simulink model "USV"  (R2022a)
settings: Solver=ode4  StartTime=0.0  StopTime=inf  FixedStep=0.001  RelTol=1e-3
PreLoadFcn:
  | [filepath,name,ext]  = fileparts(get_param(bdroot, 'FileName'));
  | InitFileName=[name,'_init.m'];
  | cd(filepath);
InitFcn:
  | [filepath,name,ext]  = fileparts(get_param(bdroot, 'FileName'));
  | InitFileName=[name,'_init.m'];
  | cd(filepath);
  | try
  | run(InitFileName);
  | end
values from neighbouring files (symbols this model uses):
  BoatParam_cf = 0.1    [USV_init.m]
  BoatParam_cg = 0.1    [USV_init.m]
  BoatParam_len = 1.5    [USV_init.m]
  BoatParam_lenSlope = pi/6    (= 0.523598775598)    [USV_init.m]
  BoatParam_waterDensity = 1000    [USV_init.m]
  BoatParam_widSlope = pi/4    (= 0.785398163397)    [USV_init.m]
  BoatParam_width = 0.8    [USV_init.m]
  ModelPara_coborigin = [0;0;0]    [USV_init.m]
  ModelParam_envAltitude = -600    [USV_init.m]
  ModelParam_GPSEphFinal = 0.3    [USV_init.m]
  ModelParam_GPSEpvFinal = 0.4    [USV_init.m]
  ModelParam_noiseGPSSampTime = 0.2    [USV_init.m]
  ModelParam_noisePowerOffGainAccel = 0.04    [USV_init.m]
  ModelParam_noisePowerOffGainAccelZ = 0.03    [USV_init.m]
  ModelParam_noisePowerOffGainGyro = 0.02    [USV_init.m]
  ModelParam_noisePowerOffGainGyroZ = 0.025    [USV_init.m]
  ModelParam_noisePowerOffGainMag = 0.02    [USV_init.m]
  ModelParam_noisePowerOffGainMagZ = 0.035    [USV_init.m]
  ModelParam_noisePowerOnGainAccel = 0.8    [USV_init.m]
  ModelParam_noisePowerOnGainAccelZ = 4.5    [USV_init.m]
  ModelParam_noisePowerOnGainGyro = 2    [USV_init.m]
  ModelParam_noisePowerOnGainGyroZ = 1    [USV_init.m]
  ModelParam_noisePowerOnGainMag = 0.025    [USV_init.m]
  ModelParam_noisePowerOnGainMagZ = 0.05    [USV_init.m]
  ModelParam_noiseUpperGPS = 0.5    [USV_init.m]
  ModelParam_uavCCm = [1 1 1]*200    [USV_init.m]
  ModelParam_uavCd = [2 200 200]    [USV_init.m]
  ModelParam_uavDearo = -0    (= 0)    [USV_init.m]
  ModelParam_uavMass = 227    [USV_init.m]
  ModelParam_uavType = int16(608)    [USV_init.m]
  motor = [motor,motorTmp]    [USV_init.m]
undefined symbols (not defined in the file or in its folder): Earth, ModelParam_GPSEpvInitial, ModelParam_GPSEpvTimeConstant, ModelParam_timeSamp, Newton, Raphson, USVPara, WGS84
libraries: RflySimModelLab x8, FaultUSVModelLib x4, aerolibtransform2 x4, vrlib x4, sharedutil x3, aerolibasang x3, sharedtransform x2, shared6dof x1, aerolibatmos2 x1, aerolibconvert2 x1, aerolibobsolete x1, simulink x1
(part 1 of 2)
settings Model: SimulationMode=accelerator  Creator=Jinrui  LastModifiedBy=dream
settings SolverCC: AlgebraicLoopSolver=TrustRegion
settings DataIOCC: ReturnWorkspaceOutputs=off
settings OptimizationCC: ZeroExternalMemoryAtStartup=off  ZeroInternalMemoryAtStartup=off  EfficientTunableParamExpr=on
settings DebuggingCC: ParameterTunabilityLossMsg=error  UnconnectedInputMsg=warning  UnconnectedOutputMsg=warning  UnconnectedLineMsg=warning  SFMachineParentedDataDiag=warning  ArithmeticOperatorsInVariantConditions=warning
settings SFSimCC: SimUseLocalCustomCode=off  MATLABDynamicMemAlloc=off  CustomCodeUndefinedFunction=UseInterfaceOnly  SimTargetLang=C++
settings RTWCC: SystemTargetFile=ert.tlc  GenCodeOnly=on  GenerateMakefile=off  PackageGeneratedCodeAndArtifacts=on  PackageName=MulticopterModel  TemplateMakefile=ert_default_tmf  RTWUseLocalCustomCode=off  TargetLang=C++  RTWCompilerOptimization=on
settings CodeAppCC: ForceParamTrailComments=on  OperatorAnnotations=on  SimulinkDataObjDesc=on  SFDataObjDesc=on  MATLABFcnDesc=on  InsertBlockDesc=on  StateflowObjectComments=on  MATLABSourceComments=on
settings ERTTargetCC: TargetLangStandard=C++03 (ISO)  MultiwordLength=2048  GenerateSampleERTMain=on  CodeInterfacePackaging=C++ class  SupportContinuousTime=on  MultiInstanceErrorCode=None  RootIOFormat=Structure reference  ERTCustomFileTemplate=example_file_process.tlc  ERTFilePackagingFormat=Compact
settings SimscapeCC: SimscapeNormalizeSystem=off

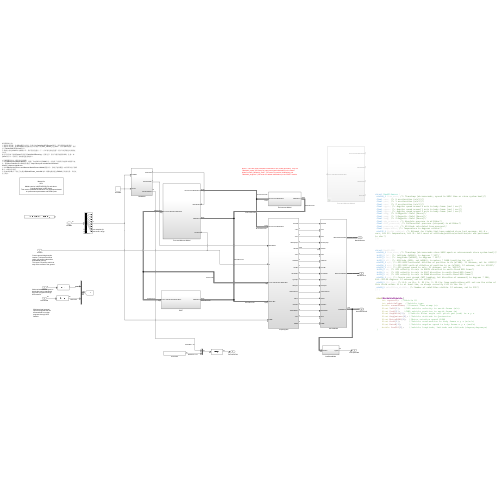
[thumbnail: Simulink's stored preview of the top-level diagram]
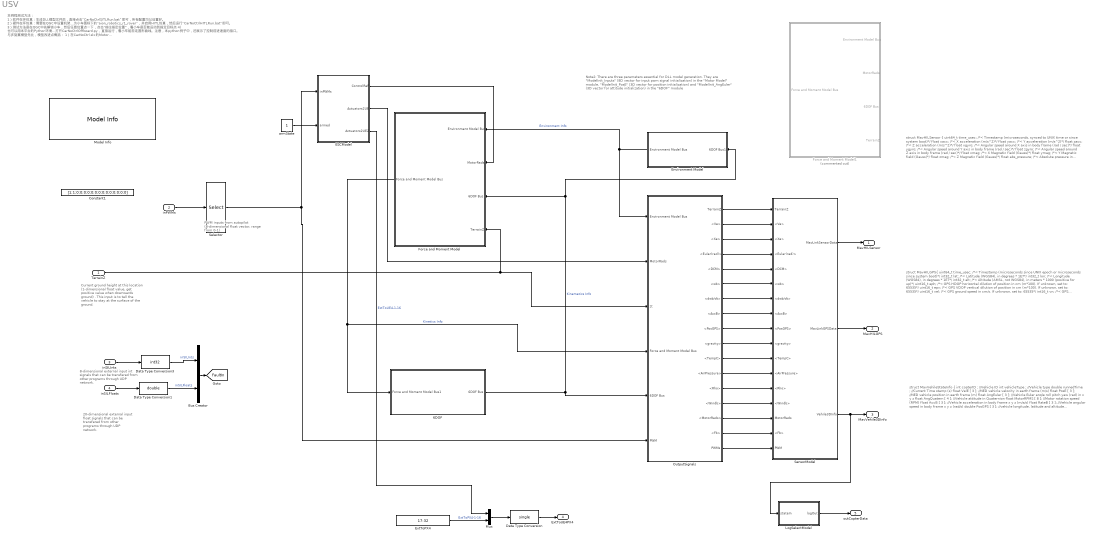
== system USV ==
  note: PWM inputs from autopilot (8-dimensional float vector, range from 0-1)
  note: Note2: There are three parameters essential for DLL model generation. They are "ModelInit_Inputs" (8D vector for input pwm signal initialization) in the "Motor Model" module, "ModelInit_PosE" (3D vector for position initialization) and "ModelInit_AngEuler" (3D vector for attitude initialization) in the "6DOF" module
  note: Current ground height at this location (1-dimensional float value, get positive value when downwards ground) .
      | This input is to tell the vehicle to stay at the surface of the ground.
  note: 本例程测试方法：
      | 1）软件在环仿真：生成DLL模型文件后，直接点击“CarNoCtrlSITLRun.bat”即可，所有配置均以设置好。
      | 2）硬件在环仿真：需要在QGC中设置机架为小车图标下的“aion_robotics_r1_rover”，并启用HITL仿真，然后运行“CarNoCtrlHITLRun.bat”即可。
      | 3）测试方法是在QGC中先解锁小车，然后任意位置点一下，点击"前往指定位置"，看小车是否能运动到指定目标点
      | 4) 也可以用本平台的Python环境打开CarNoCtrlOffboard.py，直接运行，看小车能否走圆形曲线。注意，本python例子中，还展示了控制前进速度的接口。
      |
      | 与多旋翼模型先比，模型改进点概括：
      | 1）在CarNoCtrl.slx的Motor Model中，设置了只响应0和1号PWM信号，分别给了左侧两个电机和右侧两个电机，遵循Aion Robotics R1 UGV机架模式。https://docs.px4.io/master/en/airframes/airframe_reference.html#rover
      | 2）在CarNoCtrl.slx的Force and Moment Model/Ground Model模型中个，修改了地面模型，响应四个轮子的摩擦力，来驱动车前进。
      | 3）在init.m参数中，设定了电机参数ModelParam_motorWb为0，确保电机转速与PWM成正比例关系，从而支持正反转。
  note: struct MavHILGPS{
      | uint64_t time_usec; /*< Timestamp (microseconds since UNIX epoch or microseconds since system boot)*/
      | int32_t lat; /*< Latitude (WGS84), in degrees * 1E7*/
      | int32_t lon; /*< Longitude (WGS84), in degrees * 1E7*/
      | int32_t alt; /*< Altitude (AMSL, not WGS84), in meters * 1000 (positive for up)*/
      | uint16_t eph; /*< GPS HDOP horizontal dilution of position in cm (m*100). If unknown, set to: 65535*/
      | uint16_t epv; /*< GPS VDOP vertical dilution of position in cm (m*100). If unknown, set to: 65535*/
      | uint16_t vel; /*< GPS ground speed in cm/s. If unknown, set to: 65535*/
      | int16_t vn; /*< GPS velocity in cm/s in NORTH direction in earth-fixed NED frame*/
      | int16_t ve; /*< GPS velocity in cm/s in EAST direction in earth-fixed NED frame*/
      | int16_t vd; /*< GPS velocity in cm/s in DOWN direction in earth-fixed NED frame*/
      | uint16_t cog; /*< Course over ground (NOT heading, but direction of movement) in degrees * 100, 0.0..359.99 degrees. If unknown, set to: 65535*/
      | uint8_t fix_type; /*< 0-1: no fix, 2: 2D fix, 3: 3D fix. Some applications will not use the value of this field unless it is at least two, so always correctly fill in the fix.*/
      | uint8_t satellites_visible; /*< Number of satellites visible. If unknown, set to 255*/
      | }) ;
  note: struct MavHILSensor {
      | uint64_t time_usec; /*< Timestamp (microseconds, synced to UNIX time or since system boot)*/
      | float xacc; /*< X acceleration (m/s^2)*/
      | float yacc; /*< Y acceleration (m/s^2)*/
      | float zacc; /*< Z acceleration (m/s^2)*/
      | float xgyro; /*< Angular speed around X axis in body frame (rad / sec)*/
      | float ygyro; /*< Angular speed around Y axis in body frame (rad / sec)*/
      | float zgyro; /*< Angular speed around Z axis in body frame (rad / sec)*/
      | float xmag; /*< X Magnetic field (Gauss)*/
      | float ymag; /*< Y Magnetic field (Gauss)*/
      | float zmag; /*< Z Magnetic field (Gauss)*/
      | float abs_pressure; /*< Absolute pressure in millibar*/
      | float diff_pressure; /*< Differential pressure (airspeed) in millibar*/
      | float pressure_alt; /*< Altitude calculated from pressure*/
      | float temperature; /*< Temperature in degrees celsius*/
      | uint32_t fields_updated; /*< Bitmask for fields that have updated since last message, bit 0 = xacc, bit 12: temperature, bit 31: full reset of attitude/position/velocities/etc was performed in sim.*/
      | });
  note: struct MavVehileStateInfo {
      | int copterID ; //Vehicle ID
      | int vehicleType ; //Vehicle type
      | double runnedTime ; //Current Time stamp (s)
      | float VelE [ 3 ]; //NED vehicle velocity in earth frame (m/s)
      | float PosE [ 3 ]; //NED vehicle position in earth frame (m)
      | float AngEuler [ 3 ]; //Vehicle Euler angle roll pitch yaw (rad) in x y z
      | float AngQuatern [ 4 ]; //Vehicle attitude in Quaternion
      | float MotorRPMS [ 8 ]; //Motor rotation speed (RPM)
      | float AccB [ 3 ]; //Vehicle acceleration in body frame x y z (m/s/s)
      | float RateB [ 3 ]; //Vehicle angular speed in body frame x y z (rad/s)
      | double PosGPS [ 3 ]; //vehicle longitude, latitude and altitude (degree,degree,m)
      | }
  note: 20-dimensional external input float signals that can be transfered from other programs through UDP network.
  note: 8-dimensional external input int signals that can be transfered from other programs through UDP network.
  TerrainZ : Inport
  inPWMs : Inport  Port=2
  inSILInts : Inport  Port=3  OutDataTypeStr=int32  PortDimensions=8
  inSILFloats : Inport  Port=4  OutDataTypeStr=single  PortDimensions=20
  6DOF : Subsystem
  Bus Creator : BusCreator  Inputs=2
  Constant1 : Constant  Value=[1;1;0;0;0;0;0;0;0;0;0;0;0;0;0;0]
  Data Type Conversion : DataTypeConversion  OutDataTypeStr=single  SaturateOnIntegerOverflow=off  RndMeth=Floor
  Data Type Conversion1 : DataTypeConversion  OutDataTypeStr=double  SaturateOnIntegerOverflow=off  RndMeth=Floor
  Data Type Conversion3 : DataTypeConversion  OutDataTypeStr=int32  SaturateOnIntegerOverflow=off  RndMeth=Floor
  ESCModel : Subsystem
  Environment Model : Subsystem
  ExtToPX4 : Constant  Value=17:32
  Force and Moment Model : Subsystem
  Force and Moment Model1 : Subsystem  Commented=on
  LogSelectModel : Subsystem
  Model Info : simulink/Model-Wide Utilities/Model Info  Frame=on  DisplayStringWithTags=|  HorizontalTextAlignment=Center  LeftAlignmentValue=0.5
      | Model Info
      | %<ModelName> 
      | %<Description>   
      | Matlab version is MATLAB R2017b and above. 
      | Coordinate frame is NED frame.
      |  This model  simulates the behavior of a multicopters based 
      | on performance parameters and RPM inputs
  Mux : Mux  Inputs=2
  OutputSignals : Subsystem
  Selector : Selector  InputPortWidth=16  IndexOptions=Index vector (dialog)  Indices=[1:8]  OutputSizes=1
  SensorModel : Subsystem
  armState : Constant
  MavHILSensor : Outport  OutDataTypeStr=Bus: MavLinkSensor  VectorParamsAs1DForOutWhenUnconnected=off
  MavHILGPS : Outport  Port=2  OutDataTypeStr=Bus: MavLinkGPS  VectorParamsAs1DForOutWhenUnconnected=off
  MavVehile3DInfo : Outport  Port=3  OutDataTypeStr=Bus: MavVehileInfo  VectorParamsAs1DForOutWhenUnconnected=off
  ExtToUE4PX4 : Outport  Port=4  OutDataTypeStr=single  PortDimensions=32  VectorParamsAs1DForOutWhenUnconnected=off
  outCopterData : Outport  Port=5  OutDataTypeStr=double  PortDimensions=32  VectorParamsAs1DForOutWhenUnconnected=off
  tag scope: FaultIn=global
  wires:
  OutputSignals/9(<PosGPS>) -> SensorModel/9(<PosGPS>)
  Environment Model/1(Environment Model Bus) -> Force and Moment Model/1(Environment Model Bus), OutputSignals/1(Environment Model Bus)  "Environment Info"
  OutputSignals/3(<Xe>) -> SensorModel/3(<Xe>)
  SensorModel/1(MavLinkSensorData) -> MavHILSensor/1
  OutputSignals/15(<MotorRads>) -> SensorModel/15(MotorRads)
  OutputSignals/12(<AirPressure>) -> SensorModel/12(<AirPressure>)
  Data Type Conversion/1 -> ExtToUE4PX4/1
  Selector/1 -> OutputSignals/6(PWM), ESCModel/1(inPWMs)
  OutputSignals/17(PWMs) -> SensorModel/17(PWM)
  OutputSignals/4(<Eular(rad)>) -> SensorModel/4(<Eular(rad)>)
  OutputSignals/2(<Ve>) -> SensorModel/2(<Ve>)
  OutputSignals/13(<Rho>) -> SensorModel/13(<Rho>)
  OutputSignals/8(<AccB>) -> SensorModel/8(<AccB>)
  SensorModel/3(Vehile3DInfo) -> LogSelectModel/1(stateIn), MavVehile3DInfo/1
  inPWMs/1 -> Selector/1
  SensorModel/2(MavLinkGPSData) -> MavHILGPS/1
  OutputSignals/16(<Fb>) -> SensorModel/16(<Fb>)
  ESCModel/2(Actuators2UE) -> OutputSignals/2(MotorRads)
  OutputSignals/1(TerrainZ) -> SensorModel/1(TerrainZ)
  TerrainZ/1 -> Force and Moment Model/4(TerrainZ), OutputSignals/3(zt)
  OutputSignals/10(<gravity>) -> SensorModel/10(<gravity>)
  OutputSignals/6(<wb>) -> SensorModel/6(<wb>)
  OutputSignals/14(<Windb>) -> SensorModel/14(<Windb>)
  OutputSignals/5(<DCM>) -> SensorModel/5(<DCM>)
  Mux/1 -> Data Type Conversion/1
  ExtToPX4/1 -> Mux/2  "ExtToPX4-1-16"
  ESCModel/1(ControlRef) -> Force and Moment Model/2(MotorRads)
  OutputSignals/11(<TempC>) -> SensorModel/11(<TempC>)
  ESCModel/3(Actuators2UE2) -> Mux/1  "ExtToUE4-1-16"
  6DOF/1(6DOF Bus) -> Environment Model/1(6DOF Bus1), Force and Moment Model/3(6DOF Bus), OutputSignals/5(6DOF Bus)  "Kinematics Info"
  OutputSignals/7(<dwb/dt>) -> SensorModel/7(<dwb/dt>)
  Force and Moment Model/1(Force and Moment Model Bus) -> OutputSignals/4(Force and Moment Model Bus), 6DOF/1(Force and Moment Model Bus1)  "Kinetics Info"
  armState/1 -> ESCModel/2(armed)
  Data Type Conversion1/1 -> Bus Creator/2  "inSILFloats"
  Bus Creator/1 -> [FaultIn]
  Data Type Conversion3/1 -> Bus Creator/1  "inSILInts"
  LogSelectModel/1(logOut) -> outCopterData/1
  inSILInts/1 -> Data Type Conversion3/1
  inSILFloats/1 -> Data Type Conversion1/1

== system USV/6DOF ==
  Force and Moment Model Bus1 : Inport
  Bus Creator : BusCreator  Inputs=8
  Bus Selector2 : BusSelector  OutputSignals=Fb,Mb
  Custom Variable Mass 6DOF (Quaternion) : shared6dof/6DOF (Euler Angles)  units=Metric (MKS)  mtype=Fixed  rep=Quaternion  xme_0=ModelInit_PosE  Vm_0=ModelInit_VelB  eul_0=ModelInit_AngEuler  pm_0=ModelInit_RateB  mass_0=ModelParam_uavMass  mass_e=0.5  mass_f=2.0  inertia=ModelParam_uavJ  inertia_e=eye(3)  inertia_f=2*eye(3)  k_quat=1.0  vre_flag=off  abi_flag=off  aMode=aMode  xme_statename=''  Vm_statename=''  eul_statename=''  quat_statename=''  pm_statename=''  mass_statename=''
      settings: SourceProductBaseCode=AE,PW,DR,MT,VE
  6DOF Bus : Outport  VectorParamsAs1DForOutWhenUnconnected=off
  wires:
  Custom Variable Mass 6DOF (Quaternion)/8 -> Bus Creator/8  "AccB"
  Custom Variable Mass 6DOF (Quaternion)/5 -> Bus Creator/5  "Vb"
  Custom Variable Mass 6DOF (Quaternion)/6 -> Bus Creator/6  "wb"
  Custom Variable Mass 6DOF (Quaternion)/1 -> Bus Creator/1  "Ve"
  Custom Variable Mass 6DOF (Quaternion)/4 -> Bus Creator/4  "DCM"
  Custom Variable Mass 6DOF (Quaternion)/2 -> Bus Creator/2  "Xe"
  Custom Variable Mass 6DOF (Quaternion)/3 -> Bus Creator/3  "Eular(rad)"
  Custom Variable Mass 6DOF (Quaternion)/7 -> Bus Creator/7  "dwb/dt"
  Bus Creator/1 -> 6DOF Bus/1
  Force and Moment Model Bus1/1 -> Bus Selector2/1
  Bus Selector2/2 -> Custom Variable Mass 6DOF (Quaternion)/2  "<Mb>"
  Bus Selector2/1 -> Custom Variable Mass 6DOF (Quaternion)/1  "<Fb>"

== system USV/ESCModel ==
  note: 这个是输出给到UE用于舵机转动显示的，因此需要调整顺序到与UE对应，且修改单位到合适值。
  note: 输出的是8维向量
  note: Ch1:roll, -1~1
      | Ch2:Pitch, -1~1
      | Ch3:throttle,-1~1
      | Ch4:rudder,-1~1
      |
      | Initial PWM: 0 0 -1 0
      | Pitch channel, low position for -1
      | throttle channel, low position for -1
      | Roll channel, left position for -1
      | rudder channel, right position for -1, so the value should be reversed
  inPWMs : Inport
  armed : Inport  Port=2
  ESC Fault : FaultUSVModelLib/ESC Fault  FaultParamStruct=ESCFault  ComParamVect=FaultParamAPI  SSRTWFcnClass=[]
  ESC_All1 : RflySimModelLab/ESC_All  ESCParam=ESC
  ToUEActuators : Subsystem
  ControlRef : Outport  VectorParamsAs1DForOutWhenUnconnected=off
  Actuators2UE : Outport  Port=2  VectorParamsAs1DForOutWhenUnconnected=off
  Actuators2UE2 : Outport  Port=3  VectorParamsAs1DForOutWhenUnconnected=off
  wires:
  inPWMs/1 -> ESC_All1/1
  armed/1 -> ESC_All1/2
  ToUEActuators/1(UERads) -> Actuators2UE/1
  ToUEActuators/2(UERads2) -> Actuators2UE2/1
  [FaultIn] -> ESC Fault/1
  ESC Fault/1 -> ControlRef/1, ToUEActuators/1(inMotorRads)
  ESC_All1/1 -> ESC Fault/2

== system USV/Environment Model ==
  6DOF Bus1 : Inport
  Bus Creator : BusCreator  Inputs=6
  Bus Selector : BusSelector  OutputSignals=Xe
  Bus Selector1 : BusSelector  OutputSignals=Windb
  Flat Earth to LLA : aerolibtransform2/Flat Earth to LLA  units=Metric (MKS)  ptype=Earth (WGS84)  F=1/298.257223563  R=6378137  refPosPort=off  LL0=ModelParam_GPSLatLong  psi=0
  ISA Atmosphere Model : aerolibatmos2/ISA Atmosphere Model  custom=off  g=9.80665  gamma=1.4  R=287.0531  L=0.0065  h_trop=11000  h_strat=20000  rho0=1.225  P0=101325  T0=288.15  h0=0
  ModelParam.envAltitude : Constant  Value=ModelParam_envAltitude
  Mux : Mux  Inputs=2
  Reshape : Reshape
  Saturation_1 : Saturate  UpperLimit=100000  LowerLimit=0
  Temperature Conversion : aerolibconvert2/Temperature Conversion  IU=K  OU=C
      settings: SourceProductBaseCode=AE
  TemperatureConstant : Constant  Value=25
  Terminator2 : Terminator
  Terminator3 : Terminator
  "WGS84 Gravity Model " : aerolibobsolete/WGS84 Gravity Model   model=WGS84 Taylor Series  units=Metric (MKS)  no_atmos=on  precessing=on  jd_loc=off  month=October  day=10  year=2004  no_centrifugal=on  action=Warning
      settings: SourceProductBaseCode=AE
  WindFault : FaultUSVModelLib/WindFault  FaultParamStruct=WindFault  ComParamVect=FaultParamAPI
  Environment Model Bus : Outport  VectorParamsAs1DForOutWhenUnconnected=off
  wires:
  "WGS84 Gravity Model "/1 -> Reshape/1
  Reshape/1 -> Bus Creator/2  "gravity"
  ISA Atmosphere Model/1 -> Temperature Conversion/1
  ISA Atmosphere Model/2 -> Terminator3/1
  ISA Atmosphere Model/3 -> Bus Creator/4  "AirPressure"
  ISA Atmosphere Model/4 -> Bus Creator/5  "Rho"
  Flat Earth to LLA/2 -> Saturation_1/1
  Saturation_1/1 -> Mux/2, ISA Atmosphere Model/1
  ModelParam.envAltitude/1 -> Flat Earth to LLA/2
  Mux/1 -> Bus Creator/1, "WGS84 Gravity Model "/1  "PosGPS"
  Flat Earth to LLA/1 -> Mux/1
  Temperature Conversion/1 -> Terminator2/1
  TemperatureConstant/1 -> Bus Creator/3  "TempC"
  6DOF Bus1/1 -> WindFault/2, Bus Selector/1
  Bus Selector/1 -> Flat Earth to LLA/1  "<Xe>"
  Bus Creator/1 -> Environment Model Bus/1
  [FaultIn] -> WindFault/1
  WindFault/1 -> Bus Selector1/1
  Bus Selector1/1 -> Bus Creator/6  "<Windb>"

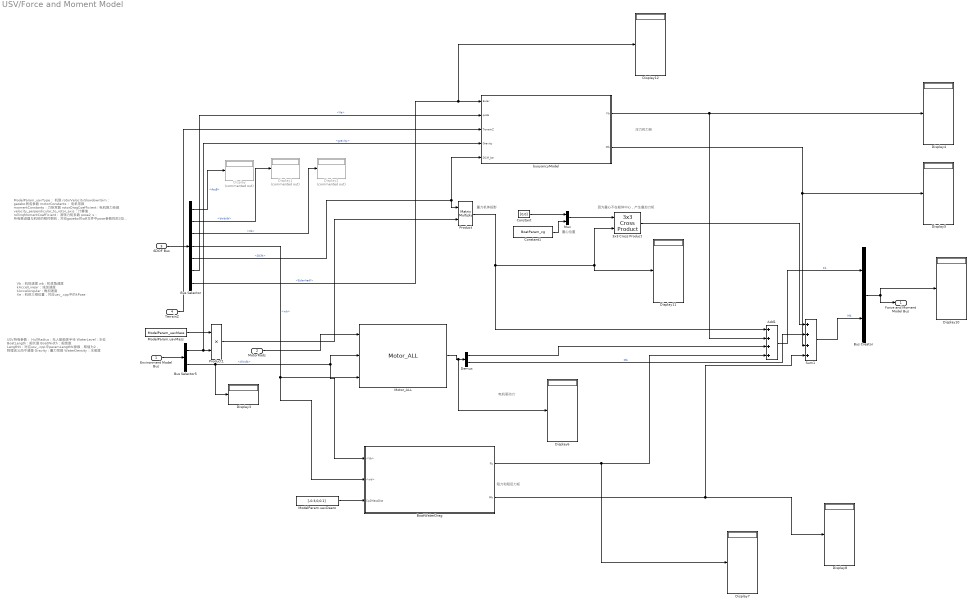
== system USV/Force and Moment Model ==
  note: 浮力和力矩
  note: 电机驱动力
  note: 重力机体投影
  note: 因为重心不在船体中心，产生叠加力矩
  note: 重心位置
  note: Vb：机体速度
      | wb：机体角速度
      | kAccelLinear ：线加速度
      | kAccelAngular：角加速度
      | Xe：机体三维位置，对应usv_.cpp中的kPose
  note: USV特有参数：
      |
      | HullRadius：无人船船体半径
      | WaterLevel：水位
      | BoatLength：船长度
      | BoatWidth：船宽度
      | LengthN：对应usv_.cpp中paramLengthN参数，取值为2， 物理含义尚不清楚
      | Gravity：重力常数
      | WaterDensity：水密度
  note: ModelParam_uavType： 机型
      | rotorVelocitySlowdownSim： gazebo同名参数
      | motorConstants： 电机常数
      | momentConstants：力矩常数
      | rotorDragCoefficient：电机阻力系数
      | velocity_perpendicular_to_rotor_axis：计算值
      |
      | rollingMomentCoefficient： 滚转力矩系数
      | pose2_s： 所有推进器与机体的相对朝向，对应gazebo的sdf文件中pose参数的后3位
      | Qua_s：推进器产生的力矩转换到机体坐标系时使用的四元数
  note: 阻力和阻尼力矩
  Environment Model Bus : Inport
  MotorRads : Inport  Port=2
  6DOF Bus : Inport  Port=3
  TerrainZ : Inport  Port=4
  3x3 Cross Product : sharedutil/3x3 Cross Product  aMode=aMode
      settings: SourceProductBaseCode=AE,PW,DR,MT,VE
  Add1 : Sum  Inputs=++++
  BoatWaterDrag : Subsystem
  Bus Creator : BusCreator  Inputs=2
  Bus Selector : BusSelector  OutputSignals=AccB,dwb/dt,Vb,wb,DCM,Xe,Eular(rad)
  Bus Selector5 : BusSelector  OutputSignals=gravity,Windb
  Constant : Constant  Value=[0,0]
  Constant1 : Constant  Value=BoatParam_cg
  Demux : Demux  Outputs=2
  Display : Display  Commented=on
  Display1 : Display  Commented=on
  Display{3..8,10..12} (9 alike) : Display
  Display2 : Display  Commented=on
  ModelParam.uavDearo : Constant  Value=[-0.3,0,0.1]
  ModelParam.uavMass : Constant  Value=ModelParam_uavMass
  Motor_ALL : RflySimModelLab/Motor_ALL  MotorParam=motor
  Mux : Mux  Inputs=2
  Product : Product  Multiplication=Matrix(*)
  Product1 : Product
  Sum1 : Sum  Inputs=++++
  buoyancyModel : Subsystem
  Force and Moment Model Bus : Outport  VectorParamsAs1DForOutWhenUnconnected=off
  wires:
  Bus Selector5/1 -> buoyancyModel/4(Gravity), Product1/2  "<gravity>"
  ModelParam.uavMass/1 -> Product1/1
  Environment Model Bus/1 -> Bus Selector5/1
  Bus Selector/5 -> buoyancyModel/5(DCM_be), Product/1  "<DCM>"
  Bus Selector5/2 -> Display3/1, BoatWaterDrag/1(<Vb>), Motor_ALL/2  "<Windb>"
  Bus Selector/1 -> Display/1  "<AccB>"
  Bus Selector/6 -> buoyancyModel/2(posE)  "<Xe>"
  Bus Selector/4 -> BoatWaterDrag/2(<wb>), Motor_ALL/3  "<wb>"
  Bus Selector/2 -> Display1/1  "<dwb/dt>"
  Bus Selector/3 -> Display2/1  "<Vb>"
  Constant1/1 -> Mux/2
  Constant/1 -> Mux/1
  Bus Creator/1 -> Force and Moment Model Bus/1, Display10/1
  Demux/1 -> Add1/3
  6DOF Bus/1 -> Bus Selector/1
  Sum1/1 -> Bus Creator/2  "Mb"
  Add1/1 -> Bus Creator/1  "Fb"
  Product1/1 -> Product/2
  Product/1 -> Display11/1, 3x3 Cross Product/2, Add1/1
  Demux/2 -> Sum1/2  "Mb"
  TerrainZ/1 -> buoyancyModel/3(TerrainZ)
  ModelParam.uavDearo/1 -> BoatWaterDrag/3(Cp2MassDist)
  Bus Selector/7 -> Display12/1, buoyancyModel/1(Euler)  "<Eular(rad)>"
  Mux/1 -> 3x3 Cross Product/1
  3x3 Cross Product/1 -> Sum1/1
  buoyancyModel/1(Fb) -> Add1/2, Display4/1
  BoatWaterDrag/1(Fb) -> Display7/1, Add1/4
  BoatWaterDrag/2(Mb) -> Sum1/4, Display8/1
  buoyancyModel/2(Mb) -> Display5/1, Sum1/3
  MotorRads/1 -> Motor_ALL/1
  Motor_ALL/1 -> Display6/1, Demux/1

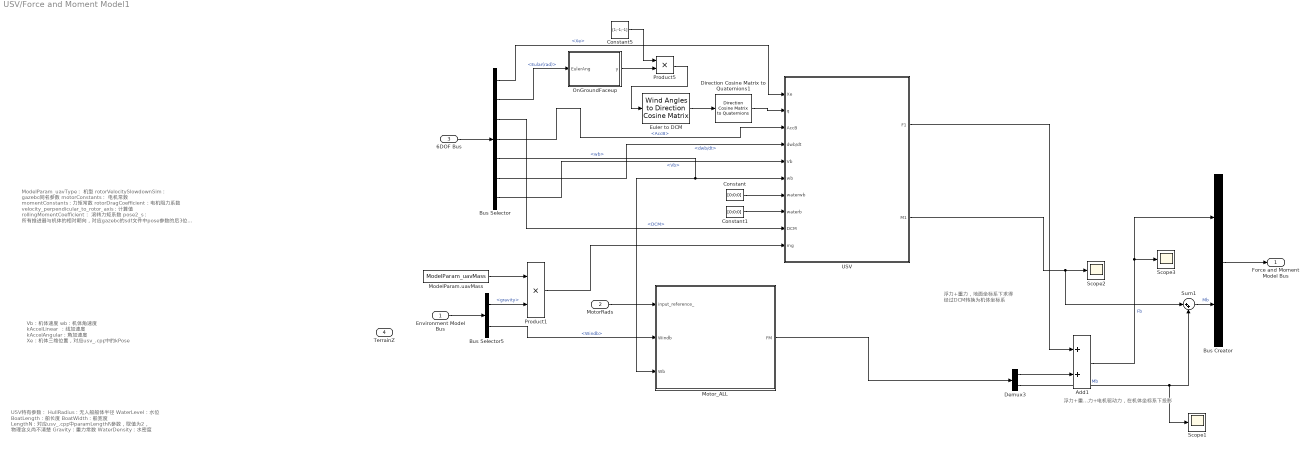
== system USV/Force and Moment Model1 ==
  note: Vb：机体速度
      | wb：机体角速度
      | kAccelLinear ：线加速度
      | kAccelAngular：角加速度
      | Xe：机体三维位置，对应usv_.cpp中的kPose
  note: USV特有参数：
      |
      | HullRadius：无人船船体半径
      | WaterLevel：水位
      | BoatLength：船长度
      | BoatWidth：船宽度
      | LengthN：对应usv_.cpp中paramLengthN参数，取值为2， 物理含义尚不清楚
      | Gravity：重力常数
      | WaterDensity：水密度
  note: ModelParam_uavType： 机型
      | rotorVelocitySlowdownSim： gazebo同名参数
      | motorConstants： 电机常数
      | momentConstants：力矩常数
      | rotorDragCoefficient：电机阻力系数
      | velocity_perpendicular_to_rotor_axis：计算值
      |
      | rollingMomentCoefficient： 滚转力矩系数
      | pose2_s： 所有推进器与机体的相对朝向，对应gazebo的sdf文件中pose参数的后3位
      | Qua_s：推进器产生的力矩转换到机体坐标系时使用的四元数
  note: 浮力+重力+电机驱动力，在机体坐标系下投影
  note: 浮力+重力，地面坐标系下求得
      | 经过DCM转换为机体坐标系
  Environment Model Bus : Inport
  MotorRads : Inport  Port=2
  6DOF Bus : Inport  Port=3
  TerrainZ : Inport  Port=4
  Add1 : Sum
  Bus Creator : BusCreator  Inputs=2
  Bus Selector : BusSelector  OutputSignals=Xe,Eular(rad),DCM,AccB,wb,dwb/dt,Vb
  Bus Selector5 : BusSelector  OutputSignals=gravity,Windb
  Constant : Constant  Value=[0;0;0]
  Constant1 : Constant  Value=[0;0;0]
  Constant5 : Constant  Value=[1;-1;-1]
  Demux3 : Demux  Outputs=2
  Direction Cosine Matrix to Quaternions1 : sharedtransform/Direction Cosine Matrix  to Quaternions  aMode=aMode  action=None  tolerance=eps(2)
      settings: SourceProductBaseCode=AE,PW,DR,MT,VE
  Euler to DCM : aerolibtransform2/Wind Angles to  Direction Cosine Matrix
      settings: SourceProductBaseCode=AE
  ModelParam.uavMass : Constant  Value=ModelParam_uavMass
  Motor_ALL : Subsystem  AncestorBlock=RflySimModelLab/Motor_ALL  mask{MotorParam=motor}
      mask prompts: MotorParam "电机参数"
  OnGroundFaceup : MATLAB Function  TreatAsAtomicUnit=on
  Product1 : Product
  Product5 : Product
  Scope1 : Scope
  Scope2 : Scope
  Scope3 : Scope
  Sum1 : Sum  Inputs=|++
  USV : Subsystem  mask{ModelUSVPara=USVPara}
      mask prompts: ModelUSVPara "水面无人艇模型参数"
  Force and Moment Model Bus : Outport  VectorParamsAs1DForOutWhenUnconnected=off
  wires:
  Bus Selector5/1 -> Product1/2  "<gravity>"
  ModelParam.uavMass/1 -> Product1/1
  Bus Selector/2 -> OnGroundFaceup/1(EulerAng)  "<Eular(rad)>"
  Environment Model Bus/1 -> Bus Selector5/1
  Direction Cosine Matrix to Quaternions1/1 -> USV/2(q)
  Bus Selector/3 -> USV/9(DCM)  "<DCM>"
  OnGroundFaceup/1(y) -> Product5/2
  Product5/1 -> Euler to DCM/1
  Euler to DCM/1 -> Direction Cosine Matrix to Quaternions1/1
  MotorRads/1 -> Motor_ALL/1(input_reference_)
  Bus Selector5/2 -> Motor_ALL/2(Windb)  "<Windb>"
  Product1/1 -> USV/10(mg)
  Bus Selector/4 -> USV/3(AccB)  "<AccB>"
  Bus Selector/1 -> USV/1(Xe)  "<Xe>"
  Bus Selector/5 -> USV/6(wb), Motor_ALL/3(Wb)  "<wb>"
  Bus Selector/6 -> USV/4(dwb/dt)  "<dwb/dt>"
  Bus Selector/7 -> USV/5(Vb)  "<Vb>"
  Constant1/1 -> USV/8(waterb)
  Constant/1 -> USV/7(waterwb)
  Constant5/1 -> Product5/1
  Demux3/2 -> Scope1/1, Sum1/2  "Mb"
  USV/2(M1) -> Sum1/1, Scope2/1
  Sum1/1 -> Bus Creator/2  "Mb"
  Bus Creator/1 -> Force and Moment Model Bus/1
  USV/1(F1) -> Add1/1
  Motor_ALL/1(FM) -> Demux3/1
  Add1/1 -> Scope3/1, Bus Creator/1  "Fb"
  Demux3/1 -> Add1/2
  6DOF Bus/1 -> Bus Selector/1

== system USV/LogSelectModel ==
  note: 1:3
  note: 4:6
  note: 7:9
  note: 10:17
  stateIn : Inport
  Bus Selector : BusSelector  OutputSignals=AccB,RateB,VelE,MotorRPMS
  Constant : Constant  Value=[0,0,0,0,0,0,0,0,0,0,0,0,0,0,0]  OutDataTypeStr=double
  Data Type Conversion{,1..3} (4 alike) : DataTypeConversion  OutDataTypeStr=double  SaturateOnIntegerOverflow=off  RndMeth=Floor
  Mux12 : Mux  Inputs=5
  logOut : Outport
  wires:
  stateIn/1 -> Bus Selector/1
  Bus Selector/1 -> Data Type Conversion/1  "<AccB>"
  Bus Selector/2 -> Data Type Conversion1/1  "<RateB>"
  Bus Selector/3 -> Data Type Conversion2/1  "<VelE>"
  Data Type Conversion/1 -> Mux12/1
  Data Type Conversion1/1 -> Mux12/2
  Data Type Conversion2/1 -> Mux12/3
  Data Type Conversion3/1 -> Mux12/4
  Mux12/1 -> logOut/1
  Bus Selector/4 -> Data Type Conversion3/1  "<MotorRPMS>"
  Constant/1 -> Mux12/5

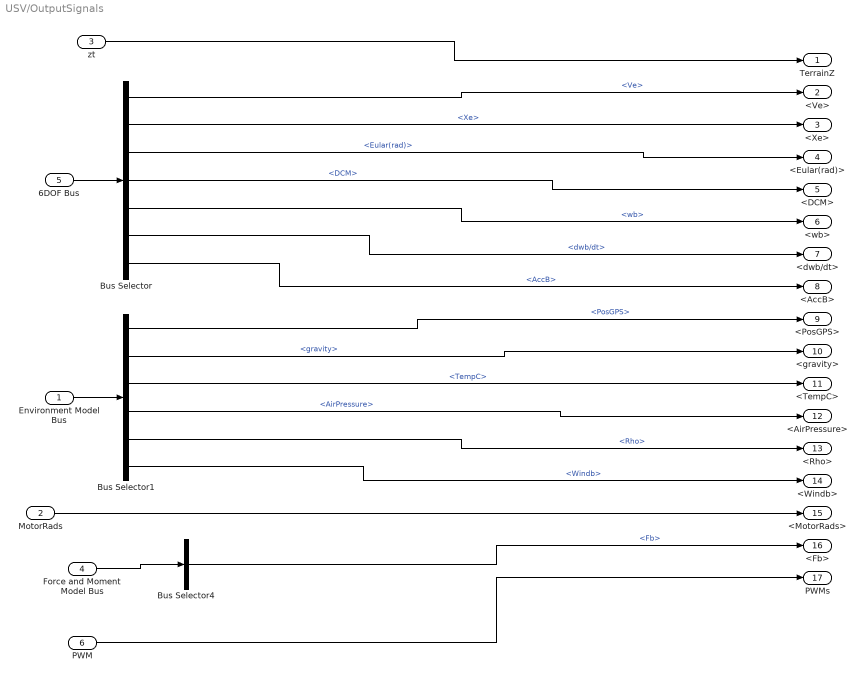
== system USV/OutputSignals ==
  Environment Model Bus : Inport
  MotorRads : Inport  Port=2
  zt : Inport  Port=3
  Force and Moment Model Bus : Inport  Port=4
  6DOF Bus : Inport  Port=5
  PWM : Inport  Port=6
  Bus Selector : BusSelector  OutputSignals=Ve,Xe,Eular(rad),DCM,wb,dwb/dt,AccB
  Bus Selector1 : BusSelector  OutputSignals=PosGPS,gravity,TempC,AirPressure,Rho,Windb
  Bus Selector4 : BusSelector  OutputSignals=Fb
  TerrainZ : Outport  VectorParamsAs1DForOutWhenUnconnected=off
  <Ve> : Outport  Port=2  VectorParamsAs1DForOutWhenUnconnected=off
  <Xe> : Outport  Port=3  VectorParamsAs1DForOutWhenUnconnected=off
  <Eular(rad)> : Outport  Port=4  VectorParamsAs1DForOutWhenUnconnected=off
  <DCM> : Outport  Port=5  VectorParamsAs1DForOutWhenUnconnected=off
  <wb> : Outport  Port=6  VectorParamsAs1DForOutWhenUnconnected=off
  <dwb/dt> : Outport  Port=7  VectorParamsAs1DForOutWhenUnconnected=off
  <AccB> : Outport  Port=8  VectorParamsAs1DForOutWhenUnconnected=off
  <PosGPS> : Outport  Port=9  VectorParamsAs1DForOutWhenUnconnected=off
  <gravity> : Outport  Port=10  VectorParamsAs1DForOutWhenUnconnected=off
  <TempC> : Outport  Port=11  VectorParamsAs1DForOutWhenUnconnected=off
  <AirPressure> : Outport  Port=12  VectorParamsAs1DForOutWhenUnconnected=off
  <Rho> : Outport  Port=13  VectorParamsAs1DForOutWhenUnconnected=off
  <Windb> : Outport  Port=14  VectorParamsAs1DForOutWhenUnconnected=off
  <MotorRads> : Outport  Port=15  VectorParamsAs1DForOutWhenUnconnected=off
  <Fb> : Outport  Port=16  VectorParamsAs1DForOutWhenUnconnected=off
  PWMs : Outport  Port=17  VectorParamsAs1DForOutWhenUnconnected=off
  wires:
  Force and Moment Model Bus/1 -> Bus Selector4/1
  MotorRads/1 -> <MotorRads>/1
  Bus Selector1/4 -> <AirPressure>/1  "<AirPressure>"
  Bus Selector/3 -> <Eular(rad)>/1  "<Eular(rad)>"
  Bus Selector1/6 -> <Windb>/1  "<Windb>"
  Bus Selector1/2 -> <gravity>/1  "<gravity>"
  PWM/1 -> PWMs/1
  Bus Selector/4 -> <DCM>/1  "<DCM>"
  Bus Selector/6 -> <dwb/dt>/1  "<dwb/dt>"
  Bus Selector1/1 -> <PosGPS>/1  "<PosGPS>"
  Bus Selector4/1 -> <Fb>/1  "<Fb>"
  Bus Selector/7 -> <AccB>/1  "<AccB>"
  Bus Selector/1 -> <Ve>/1  "<Ve>"
  Bus Selector/5 -> <wb>/1  "<wb>"
  Bus Selector/2 -> <Xe>/1  "<Xe>"
  Bus Selector1/5 -> <Rho>/1  "<Rho>"
  zt/1 -> TerrainZ/1
  Bus Selector1/3 -> <TempC>/1  "<TempC>"
  Environment Model Bus/1 -> Bus Selector1/1
  6DOF Bus/1 -> Bus Selector/1

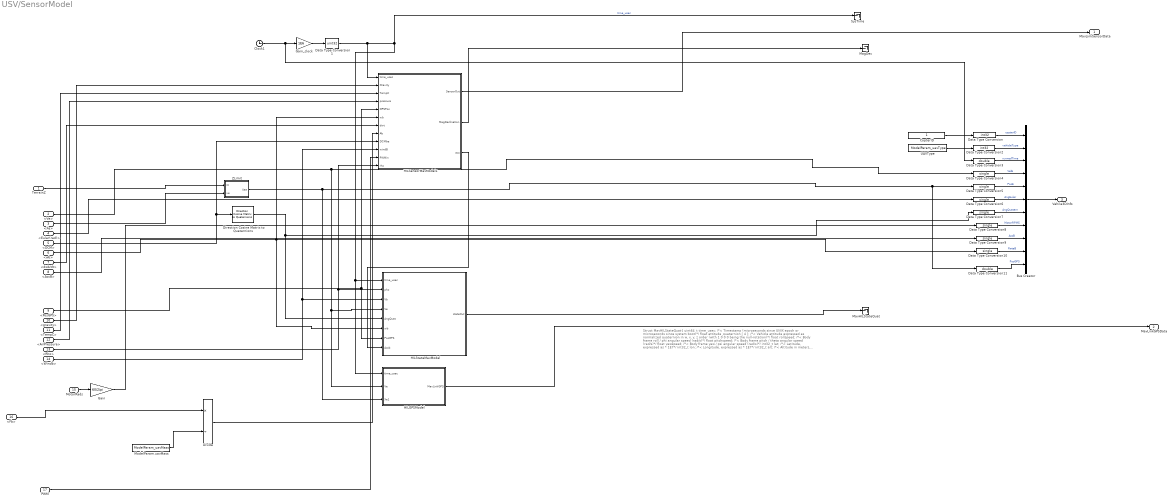
== system USV/SensorModel ==
  note: Struct MavHILStateQuat{
      | uint64_t time_usec; /*< Timestamp (microseconds since UNIX epoch or microseconds since system boot)*/
      | float attitude_quaternion [ 4 ]; /*< Vehicle attitude expressed as normalized quaternion in w, x, y, z order (with 1 0 0 0 being the null-rotation)*/
      | float rollspeed; /*< Body frame roll / phi angular speed (rad/s)*/
      | float pitchspeed; /*< Body frame pitch / theta angular speed (rad/s)*/
      | float yawspeed; /*< Body frame yaw / psi angular speed (rad/s)*/
      | int32_t lat; /*< Latitude, expressed as * 1E7*/
      | int32_t lon; /*< Longitude, expressed as * 1E7*/
      | int32_t alt; /*< Altitude in meters, expressed as * 1000 (millimeters)*/
      | int16_t vx; /*< Ground X Speed (Latitude), expressed as cm/s*/
      | int16_t vy; /*< Ground Y Speed (Longitude), expressed as cm/s*/
      | int16_t vz; /*< Ground Z Speed (Altitude), expressed as cm/s*/
      | uint16_t ind_airspeed; /*< Indicated airspeed, expressed as cm/s*/
      | uint16_t true_airspeed; /*< True airspeed, expressed as cm/s*/
      | int16_t xacc; /*< X acceleration (mg)*/
      | int16_t yacc; /*< Y acceleration (mg)*/
      | int16_t zacc; /*< Z acceleration (mg)*/
      | };
  TerrainZ : Inport
  <Ve> : Inport  Port=2
  <Xe> : Inport  Port=3
  <Eular(rad)> : Inport  Port=4
  <DCM> : Inport  Port=5
  <wb> : Inport  Port=6
  <dwb/dt> : Inport  Port=7
  <AccB> : Inport  Port=8
  <PosGPS> : Inport  Port=9
  <gravity> : Inport  Port=10
  <TempC> : Inport  Port=11
  <AirPressure> : Inport  Port=12
  <Rho> : Inport  Port=13
  <Windb> : Inport  Port=14
  MotorRads : Inport  Port=15
  <Fb> : Inport  Port=16
  PWM : Inport  Port=17
  Bus Creator : BusCreator  Inputs=11  OutDataTypeStr=Bus: MavVehileInfo
  Clock1 : Clock
  CopterID : Constant
  Data Type Conversion : DataTypeConversion  OutDataTypeStr=int32  SaturateOnIntegerOverflow=off  RndMeth=Floor
  Data Type Conversion1 : DataTypeConversion  OutDataTypeStr=uint32  SaturateOnIntegerOverflow=off  RndMeth=Floor
  Data Type Conversion{4..10} (7 alike) : DataTypeConversion  OutDataTypeStr=single  SaturateOnIntegerOverflow=off  RndMeth=Floor
  Data Type Conversion11 : DataTypeConversion  OutDataTypeStr=double  SaturateOnIntegerOverflow=off  RndMeth=Floor
  Data Type Conversion2 : DataTypeConversion  OutDataTypeStr=int32  SaturateOnIntegerOverflow=off  RndMeth=Floor
  Data Type Conversion3 : DataTypeConversion  OutDataTypeStr=double  SaturateOnIntegerOverflow=off  RndMeth=Floor
  Direction Cosine Matrix to Quaternions : sharedtransform/Direction Cosine Matrix  to Quaternions  aMode=aMode  action=None  tolerance=eps(2)
      settings: SourceProductBaseCode=AE,PW,DR,MT,VE
  Divide : Product  Inputs=*/
  Gain : Gain  Gain=60/2/pi
  Gain_clock : Gain  Gain=1E6
  HILGPSModel : Subsystem
  HILSensorMavModel1 : Subsystem
  HILStateMavModel : Subsystem
  MagDec : Terminator
  MavHILStateQuat : Terminator
  ModelParam.uavMass : Constant  Value=ModelParam_uavMass
  SysTime : Terminator
  UAVType : Constant  Value=ModelParam_uavType
  ZLimit : MATLAB Function  TreatAsAtomicUnit=on
  MavLinkSensorData : Outport  VectorParamsAs1DForOutWhenUnconnected=off
  MavLinkGPSData : Outport  Port=2  VectorParamsAs1DForOutWhenUnconnected=off
  Vehile3DInfo : Outport  Port=3  VectorParamsAs1DForOutWhenUnconnected=off
  wires:
  <Xe>/1 -> ZLimit/2(xe)
  <PosGPS>/1 -> HILSensorMavModel1/5(GPSPos), HILStateMavModel/7(PosGPS)
  <TempC>/1 -> HILSensorMavModel1/3(TempC)
  <AirPressure>/1 -> HILSensorMavModel1/4(pressure)
  Clock1/1 -> Data Type Conversion3/1, Gain_clock/1
  Data Type Conversion1/1 -> HILSensorMavModel1/1(time_usec), SysTime/1, HILGPSModel/1(time_usec), HILStateMavModel/1(time_usec)  "time_usec"
  <gravity>/1 -> HILSensorMavModel1/2(Gravity)
  <Rho>/1 -> HILSensorMavModel1/12(rho), HILStateMavModel/2(pho)
  Gain_clock/1 -> Data Type Conversion1/1
  <DCM>/1 -> HILSensorMavModel1/9(DCMbe), Direction Cosine Matrix to Quaternions/1
  <Eular(rad)>/1 -> Data Type Conversion6/1
  <dwb/dt>/1 -> HILSensorMavModel1/7(dwt)
  <wb>/1 -> HILSensorMavModel1/6(wb), Data Type Conversion10/1, HILStateMavModel/6(wb)
  <Ve>/1 -> HILGPSModel/2(Ve), HILStateMavModel/4(Ve), Data Type Conversion4/1
  TerrainZ/1 -> ZLimit/1(zt)
  CopterID/1 -> Data Type Conversion/1
  HILSensorMavModel1/2(MagDeclination) -> MagDec/1
  <AccB>/1 -> Data Type Conversion9/1
  Divide/1 -> HILSensorMavModel1/8(Ab)
  Data Type Conversion5/1 -> Bus Creator/5  "PosE"
  Data Type Conversion7/1 -> Bus Creator/7  "AngQuatern"
  Data Type Conversion4/1 -> Bus Creator/4  "VelE"
  Data Type Conversion9/1 -> Bus Creator/9  "AccB"
  Data Type Conversion10/1 -> Bus Creator/10  "RateB"
  PWM/1 -> HILSensorMavModel1/11(PWMin)
  Data Type Conversion11/1 -> Bus Creator/11  "PosGPS"
  Data Type Conversion6/1 -> Bus Creator/6  "AngEuler"
  ZLimit/1(Xee) -> HILGPSModel/3(Xe1), Data Type Conversion11/1, Data Type Conversion5/1
  Data Type Conversion/1 -> Bus Creator/1  "copterID"
  Bus Creator/1 -> Vehile3DInfo/1
  <Fb>/1 -> Divide/1
  Gain/1 -> Data Type Conversion8/1
  HILStateMavModel/1(stateOut) -> MavHILStateQuat/1
  Data Type Conversion8/1 -> Bus Creator/8  "MotorRPMS"
  Direction Cosine Matrix to Quaternions/1 -> Data Type Conversion7/1, HILStateMavModel/5(AngQuat)
  UAVType/1 -> Data Type Conversion2/1
  Data Type Conversion3/1 -> Bus Creator/3  "runnedTime"
  HILSensorMavModel1/3(acc) -> HILStateMavModel/8(Accb)
  ModelParam.uavMass/1 -> Divide/2
  Data Type Conversion2/1 -> Bus Creator/2  "vehicleType"
  HILSensorMavModel1/1(SensorOut) -> MavLinkSensorData/1
  HILGPSModel/1(MavLinkGPS) -> MavLinkGPSData/1
  <Windb>/1 -> HILSensorMavModel1/10(windB), HILStateMavModel/3(Vb)
  MotorRads/1 -> Gain/1

== system USV/ESCModel/ToUEActuators ==
  note: 舵面加入低通滤波器，使得舵面显示更平稳
  note: UE中VTOL的定义顺序如下：
      | 1. Rudder（degree)
      | 2. Propeller Front Left（rpm）
      | 3. Propeller Front Right（rpm）
      | 4. Propeller Back Left（rpm）
      | 5. Propeller Back Right（rpm）
      | 6. Propeller Back Middle（rpm）
      | 7. Flaps Left（degree)
      | 8. Flaps Right（degree)
      |
      | 9. Aileron Left（degree)
      | 10. Aileron Right（degree)
      | 11. Elevator Left（degree)
      | 12. Elevator Right（degree)
  note: ControlRef取前8个元素的向量：
      |
      | ControlRef1：前右电机rotor0（转每分）
      | ControlRef2：后左电机rotor1（转每分）
      | ControlRef3：前左电机rotor2（转每分）
      | ControlRef4：后右电机rotor3（转每分）
      | ControlRef5：推进电机thruttle（转每分）
      | ControlRef6：left_elevon（弧度）
      | ControlRef7：right_elevon（弧度）
      | ControlRef8：elevator（弧度）
  inMotorRads : Inport
  Constant1 : Constant  Value=0
  Constant2 : Constant  Value=zeros(12,1)
  Demux : Demux  Outputs=8
  Gain1 : Gain  Gain=180/pi
  Gain2 : Gain  Gain=180/pi
  Gain3 : Gain  Gain=180/pi
  Mux : Mux  Inputs=8
  Mux1 : Mux  Inputs=5
  Transfer Fcn1 : TransferFcn  Denominator=[0.1 1]
  Transfer Fcn2 : TransferFcn  Denominator=[0.1 1]
  Transfer Fcn3 : TransferFcn  Denominator=[0.1 1]
  UERads : Outport
  UERads2 : Outport  Port=2
  wires:
  inMotorRads/1 -> Demux/1
  Mux/1 -> UERads/1
  Mux1/1 -> UERads2/1
  Demux/1 -> Mux/1
  Demux/4 -> Mux/4, Mux/5
  Demux/6 -> Transfer Fcn2/1
  Demux/7 -> Transfer Fcn1/1
  Demux/8 -> Transfer Fcn3/1
  Constant2/1 -> Mux1/5
  Demux/5 -> Mux/6
  Gain1/1 -> Mux1/1
  Transfer Fcn3/1 -> Gain3/1
  Transfer Fcn1/1 -> Gain2/1
  Transfer Fcn2/1 -> Gain1/1
  Gain2/1 -> Mux1/2
  Gain3/1 -> Mux1/4, Mux1/3
  Constant1/1 -> Mux/8, Mux/7
  Demux/2 -> Mux/2
  Demux/3 -> Mux/3

== system USV/Force and Moment Model/BoatWaterDrag ==
  note: 因为船的分浪构造，船头有保持航线方向恢复的趋势，即存在侧滑角beta反馈，产生z轴力矩，使得侧滑角取向0
  note: 船的阻力与速度方向相反，大小与速度平方成正比
  <Vb> : Inport
  <wb> : Inport  Port=2
  Cp2MassDist : Inport  Port=3
  3x3 Cross Product : sharedutil/3x3 Cross Product  Commented=on  aMode=aMode
      settings: SourceProductBaseCode=AE,PW,DR,MT,VE
  Body AeroCenter : MATLAB Function  TreatAsAtomicUnit=on
  Display{1..5} (5 alike) : Display
  Display6 : Display  Commented=on
  "Incidence, Sideslip, & Airspeed" : aerolibasang/Incidence, Sideslip, & Airspeed  Commented=on
  MATLAB Function : MATLAB Function  Commented=on  TreatAsAtomicUnit=on
  ModelParam.uavCCm : Constant  Value=ModelParam_uavCCm
  ModelParam.uavCd : Constant  Value=ModelParam_uavCd
  Sum : Sum  Inputs=|++
  USVPara_Dmat : Constant  Value=USVPara.Dmat
  Fb : Outport  VectorParamsAs1DForOutWhenUnconnected=off
  Mb : Outport  Port=2  VectorParamsAs1DForOutWhenUnconnected=off
  wires:
  Body AeroCenter/1(Fd) -> Display4/1, 3x3 Cross Product/2, Fb/1
  Cp2MassDist/1 -> 3x3 Cross Product/1
  <wb>/1 -> Body AeroCenter/1(wb)
  ModelParam.uavCd/1 -> Body AeroCenter/3(Cd)
  ModelParam.uavCCm/1 -> Body AeroCenter/4(CCm)
  "Incidence, Sideslip, & Airspeed"/2 -> MATLAB Function/1(beta)
  Body AeroCenter/2(Md) -> Sum/1, Display5/1
  "Incidence, Sideslip, & Airspeed"/3 -> Display6/1, MATLAB Function/2(V)
  "Incidence, Sideslip, & Airspeed"/1 -> Display2/1
  MATLAB Function/1(M) -> Sum/2, Display3/1
  <Vb>/1 -> Body AeroCenter/2(Vb), "Incidence, Sideslip, & Airspeed"/1, Display1/1
  USVPara_Dmat/1 -> Body AeroCenter/5(Dmat)
  Sum/1 -> Mb/1

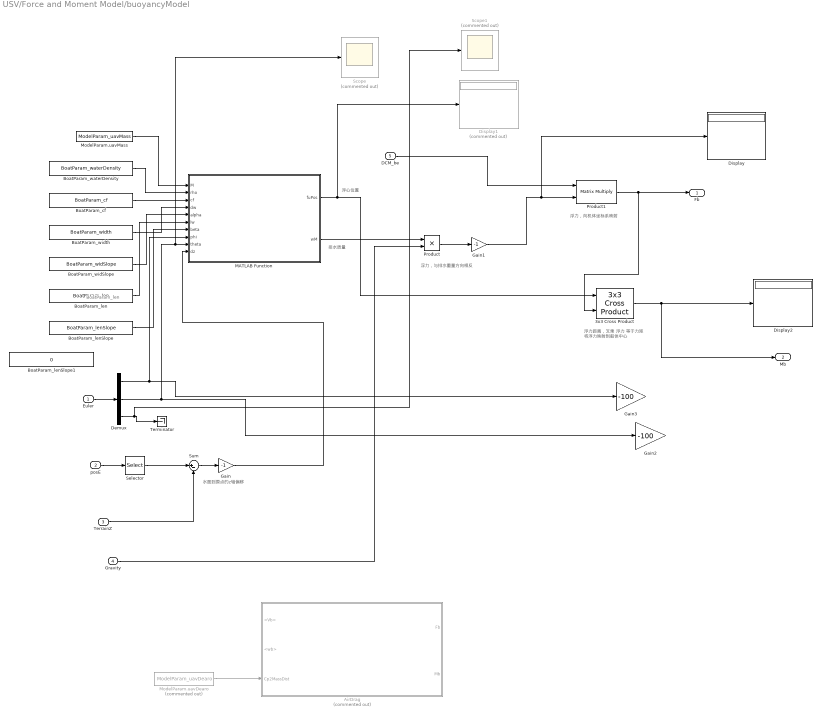
== system USV/Force and Moment Model/buoyancyModel ==
  note: 浮力距离，叉乘 浮力 等于力矩
      | 将浮力映射到船体中心
  note: 浮心位置
  note: 浮力，向机体坐标系映射
  note: 浮力，与排水重量方向相反
  note: 排水质量
  note: 水面到原点的z轴偏移
  note: BoatParam_len
  Euler : Inport
  posE : Inport  Port=2
  TerrainZ : Inport  Port=3
  Gravity : Inport  Port=4
  DCM_be : Inport  Port=5
  3x3 Cross Product : sharedutil/3x3 Cross Product  aMode=aMode
      settings: SourceProductBaseCode=AE,PW,DR,MT,VE
  AirDrag : Subsystem  Commented=on
  BoatParam_cf : Constant  Value=BoatParam_cf
  BoatParam_len : Constant  Value=BoatParam_len
  BoatParam_lenSlope : Constant  Value=BoatParam_lenSlope
  BoatParam_lenSlope1 : Constant  Value=0
  BoatParam_waterDensity : Constant  Value=BoatParam_waterDensity
  BoatParam_widSlope : Constant  Value=BoatParam_widSlope
  BoatParam_width : Constant  Value=BoatParam_width
  Demux : Demux  Outputs=3
  Display : Display
  Display1 : Display  Commented=on
  Display2 : Display
  Gain : Gain  Gain=-1
  Gain1 : Gain  Gain=-1
  Gain2 : Gain  Gain=-100
  Gain3 : Gain  Gain=-100
  MATLAB Function : MATLAB Function  TreatAsAtomicUnit=on
  ModelParam.uavDearo : Constant  Commented=on  Value=ModelParam_uavDearo
  ModelParam.uavMass : Constant  Value=ModelParam_uavMass
  Product : Product
  Product1 : Product  Multiplication=Matrix(*)
  Scope : Scope  Commented=on
  Scope1 : Scope  Commented=on
  Selector : Selector  InputPortWidth=3  IndexOptions=Index vector (dialog)  Indices=[3]  OutputSizes=1
  Sum : Sum  Inputs=|+-
  Terminator : Terminator
  Fb : Outport  VectorParamsAs1DForOutWhenUnconnected=off
  Mb : Outport  Port=2  VectorParamsAs1DForOutWhenUnconnected=off
  wires:
  3x3 Cross Product/1 -> Mb/1, Display2/1
  Euler/1 -> Demux/1
  ModelParam.uavMass/1 -> MATLAB Function/1(M)
  BoatParam_waterDensity/1 -> MATLAB Function/2(rho)
  BoatParam_cf/1 -> MATLAB Function/3(cf)
  BoatParam_width/1 -> MATLAB Function/4(dw)
  BoatParam_widSlope/1 -> MATLAB Function/5(alpha)
  BoatParam_len/1 -> MATLAB Function/6(lw)
  BoatParam_lenSlope/1 -> MATLAB Function/7(beta)
  Demux/1 -> MATLAB Function/8(phi), Gain3/1
  Demux/3 -> Scope1/1, Terminator/1
  posE/1 -> Selector/1
  Selector/1 -> Sum/1
  TerrainZ/1 -> Sum/2
  Sum/1 -> Gain/1
  Gain/1 -> MATLAB Function/10(dz)
  MATLAB Function/2(wM) -> Product/1
  Gravity/1 -> Product/2
  Product/1 -> Gain1/1
  MATLAB Function/1(fuPos) -> Display1/1, 3x3 Cross Product/1
  DCM_be/1 -> Product1/1
  Gain1/1 -> Display/1, Product1/2
  Product1/1 -> 3x3 Cross Product/2, Fb/1
  Demux/2 -> Scope/1, MATLAB Function/9(theta), Gain2/1
  ModelParam.uavDearo/1 -> AirDrag/3(Cp2MassDist)

== system USV/Force and Moment Model1/Motor_ALL ==
  input_reference_ : Inport
  Windb : Inport  Port=2
  Wb : Inport  Port=3
  Demux : Demux  Outputs=8
  Motor1 : Subsystem  AncestorBlock=RflySimModelLab/Motor  mask{MotorPara=MotorParam(1)}
      mask prompts: MotorPara "电机名"
  Motor2 : Subsystem  AncestorBlock=RflySimModelLab/Motor  mask{MotorPara=MotorParam(2)}
      mask prompts: MotorPara "电机名"
  Motor3 : RflySimModelLab/Motor  MotorPara=MotorParam(3)
  Motor4 : RflySimModelLab/Motor  MotorPara=MotorParam(4)
  Motor5 : RflySimModelLab/Motor  MotorPara=MotorParam(5)
  Motor6 : RflySimModelLab/Motor  MotorPara=MotorParam(6)
  Motor7 : RflySimModelLab/Motor  MotorPara=MotorParam(7)
  Motor8 : RflySimModelLab/Motor  MotorPara=MotorParam(8)
  Sum : Sum  Inputs=++++++++
  FM : Outport
  wires:
  Demux/8 -> Motor8/1
  Demux/7 -> Motor7/1
  Demux/6 -> Motor6/1
  Demux/5 -> Motor5/1
  Demux/4 -> Motor4/1
  Demux/3 -> Motor3/1
  Demux/2 -> Motor2/1(input_reference_)
  input_reference_/1 -> Demux/1
  Sum/1 -> FM/1
  Motor8/1 -> Sum/8
  Motor7/1 -> Sum/7
  Motor6/1 -> Sum/6
  Motor5/1 -> Sum/5
  Motor4/1 -> Sum/4
  Motor3/1 -> Sum/3
  Demux/1 -> Motor1/1(input_reference_)
  Windb/1 -> Motor1/2(Windb), Motor2/2(Windb), Motor3/2, Motor4/2, Motor5/2, Motor6/2, Motor7/2, Motor8/2
  Wb/1 -> Motor1/3(Wb), Motor2/3(Wb), Motor3/3, Motor4/3, Motor6/3, Motor8/3, Motor7/3, Motor5/3
  Motor2/1(FM) -> Sum/2
  Motor1/1(FM) -> Sum/1

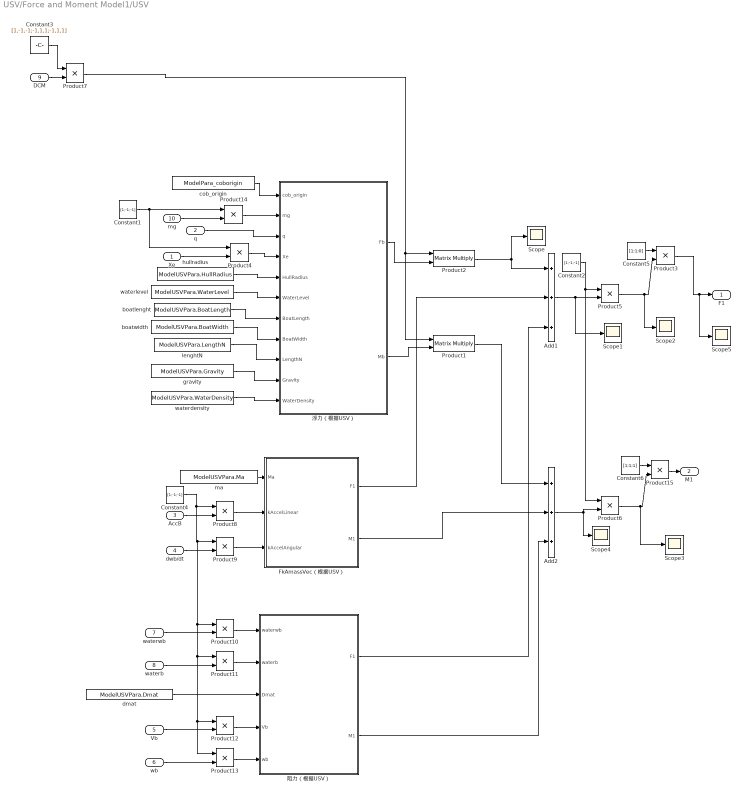
== system USV/Force and Moment Model1/USV ==
  Xe : Inport
  q : Inport  Port=2
  AccB : Inport  Port=3
  dwb/dt : Inport  Port=4
  Vb : Inport  Port=5
  wb : Inport  Port=6
  waterwb : Inport  Port=7
  waterb : Inport  Port=8
  DCM : Inport  Port=9
  mg : Inport  Port=10
  Add1 : Sum  Inputs=+++
  Add2 : Sum  Inputs=+++
  Constant1 : Constant  Value=[1;-1;-1]
  Constant2 : Constant  Value=[1;-1;-1]
  Constant3 : Constant  Value=[1,-1,-1;-1,1,1;-1,1,1]
  Constant4 : Constant  Value=[1;-1;-1]
  Constant5 : Constant  Value=[1;1;0]
  Constant6 : Constant  Value=[1;1;1]
  FkAmassVec（根据USV） : MATLAB Function  TreatAsAtomicUnit=on
  Product1 : Product  Multiplication=Matrix(*)
  Product{3..15} (13 alike) : Product
  Product2 : Product  Multiplication=Matrix(*)
  Scope{,1..5} (6 alike) : Scope
  boatlenght : Constant  Value=ModelUSVPara.BoatLength
  boatwidth : Constant  Value=ModelUSVPara.BoatWidth
  cob_origin : Constant  Value=ModelPara_coborigin
  dmat : Constant  Value=ModelUSVPara.Dmat
  gravity : Constant  Value=ModelUSVPara.Gravity
  hullradius : Constant  Value=ModelUSVPara.HullRadius
  lenghtN : Constant  Value=ModelUSVPara.LengthN
  ma : Constant  Value=ModelUSVPara.Ma
  waterdensity : Constant  Value=ModelUSVPara.WaterDensity
  waterlevel : Constant  Value=ModelUSVPara.WaterLevel
  浮力（根据USV） : MATLAB Function  TreatAsAtomicUnit=on
  阻力（根据USV） : MATLAB Function  TreatAsAtomicUnit=on
  F1 : Outport
  M1 : Outport  Port=2
  wires:
  hullradius/1 -> 浮力（根据USV）/5(HullRadius)
  waterlevel/1 -> 浮力（根据USV）/6(WaterLevel)
  boatlenght/1 -> 浮力（根据USV）/7(BoatLength)
  boatwidth/1 -> 浮力（根据USV）/8(BoatWidth)
  lenghtN/1 -> 浮力（根据USV）/9(LengthN)
  gravity/1 -> 浮力（根据USV）/10(Gravity)
  waterdensity/1 -> 浮力（根据USV）/11(WaterDensity)
  ma/1 -> FkAmassVec（根据USV）/1(Ma)
  dmat/1 -> 阻力（根据USV）/3(Dmat)
  Constant3/1 -> Product7/1
  DCM/1 -> Product7/2
  浮力（根据USV）/1(Fb) -> Product2/2
  Product7/1 -> Product1/1, Product2/1
  浮力（根据USV）/2(Mb) -> Product1/2
  Add1/1 -> Scope1/1, Product5/2
  Add2/1 -> Product6/2, Scope4/1
  Constant2/1 -> Product6/1, Product5/1
  Product6/1 -> Product15/2, Scope3/1
  FkAmassVec（根据USV）/1(F1) -> Add1/2
  阻力（根据USV）/1(F1) -> Add1/3
  FkAmassVec（根据USV）/2(M1) -> Add2/2
  阻力（根据USV）/2(M1) -> Add2/3
  q/1 -> 浮力（根据USV）/3(q)
  Xe/1 -> Product4/2
  Product4/1 -> 浮力（根据USV）/4(Xe)
  Constant4/1 -> Product13/1, Product12/1, Product11/1, Product10/1, Product9/1, Product8/1
  Product8/1 -> FkAmassVec（根据USV）/2(kAccelLinear)
  Product9/1 -> FkAmassVec（根据USV）/3(kAccelAngular)
  waterb/1 -> Product11/2
  waterwb/1 -> Product10/2
  Product10/1 -> 阻力（根据USV）/1(waterwb)
  Product11/1 -> 阻力（根据USV）/2(waterb)
  Vb/1 -> Product12/2
  wb/1 -> Product13/2
  Product12/1 -> 阻力（根据USV）/4(Vb)
  Product13/1 -> 阻力（根据USV）/5(wb)
  Product14/1 -> 浮力（根据USV）/2(mg)
  mg/1 -> Product14/2
  Constant1/1 -> Product14/1, Product4/1
  cob_origin/1 -> 浮力（根据USV）/1(cob_origin)
  AccB/1 -> Product8/2
  dwb/dt/1 -> Product9/2
  Product2/1 -> Add1/1, Scope/1
  Constant5/1 -> Product3/1
  Product5/1 -> Product3/2, Scope2/1
  Product3/1 -> Scope5/1, F1/1
  Constant6/1 -> Product15/1
  Product15/1 -> M1/1
  Product1/1 -> Add2/1

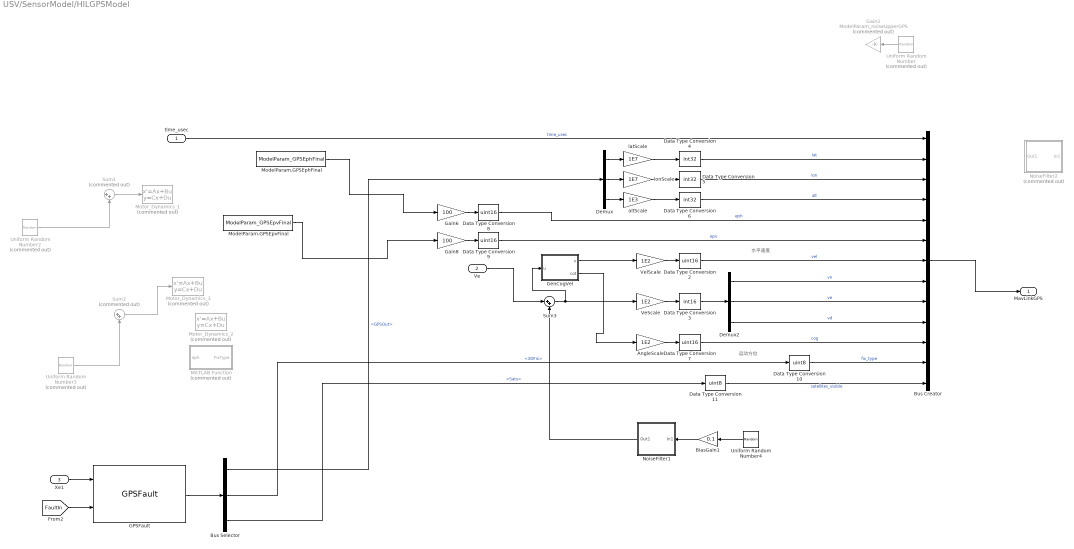
== system USV/SensorModel/HILGPSModel ==
  note: 水平速度
  note: 运动方位
  time_usec : Inport
  Ve : Inport  Port=2
  Xe1 : Inport  Port=3
  AngleScale : Gain  Gain=1E2
  BiasGain1 : Gain  Gain=0.1
  Bus Creator : BusCreator  Inputs=13  OutDataTypeStr=Bus: MavLinkGPS  NonVirtualBus=on
  Bus Selector : BusSelector  OutputSignals=GPSOut,3DFix,Sats
  Data Type Conversion10 : DataTypeConversion  OutDataTypeStr=uint8  RndMeth=Round  SaturateOnIntegerOverflow=off
  Data Type Conversion11 : DataTypeConversion  OutDataTypeStr=uint8  RndMeth=Round  SaturateOnIntegerOverflow=off
  Data Type Conversion{2,7..9} (4 alike) : DataTypeConversion  OutDataTypeStr=uint16  RndMeth=Round  SaturateOnIntegerOverflow=off
  Data Type Conversion3 : DataTypeConversion  OutDataTypeStr=int16  RndMeth=Round  SaturateOnIntegerOverflow=off
  Data Type Conversion4 : DataTypeConversion  OutDataTypeStr=int32  RndMeth=Round  SaturateOnIntegerOverflow=off
  Data Type Conversion5 : DataTypeConversion  OutDataTypeStr=int32  RndMeth=Round  SaturateOnIntegerOverflow=off
  Data Type Conversion6 : DataTypeConversion  OutDataTypeStr=int32  RndMeth=Round  SaturateOnIntegerOverflow=off
  Demux : Demux  Outputs=3
  Demux2 : Demux  Outputs=3
  GPSFault : FaultUSVModelLib/GPSFault  FaultParamStruct=SensorFault
  Gain2 : Gain  Commented=on  Gain=ModelParam_noiseUpperGPS
  Gain6 : Gain  Gain=100
  Gain8 : Gain  Gain=100
  GenCogVel : MATLAB Function  TreatAsAtomicUnit=on
  MATLAB Function : MATLAB Function  Commented=on  TreatAsAtomicUnit=on
  ModelParam.GPSEphFinal : Constant  Value=ModelParam_GPSEphFinal
  ModelParam.GPSEpvFinal : Constant  Value=ModelParam_GPSEpvFinal
  Motor_Dynamics_1 : StateSpace  Commented=on  A=-1/0.2  C=1/0.2  D=0  InitialCondition=20*0.2
  Motor_Dynamics_2 : StateSpace  Commented=on  A=-1/ModelParam_GPSEpvTimeConstant  C=1/ModelParam_GPSEpvTimeConstant  D=0  InitialCondition=ModelParam_GPSEpvInitial*ModelParam_GPSEpvTimeConstant
  Motor_Dynamics_3 : StateSpace  Commented=on  A=-1/0.2  C=1/0.2  D=0  InitialCondition=20*0.2
  NoiseFilter1 : Subsystem
  NoiseFilter2 : Subsystem  Commented=on
  Sum1 : Sum  Commented=on  Inputs=|++
  Sum2 : Sum  Commented=on  Inputs=|++
  Sum3 : Sum  Inputs=|++
  Uniform Random Number : UniformRandomNumber  Commented=on  Minimum=[-1,-1,-3]  Maximum=[1,1,3]  Seed=[14524,7875,698]  SampleTime=ModelParam_timeSamp
  Uniform Random Number2 : UniformRandomNumber  Commented=on  Minimum=-0.01  Maximum=0.01  Seed=4345454  SampleTime=ModelParam_noiseGPSSampTime
  Uniform Random Number3 : UniformRandomNumber  Commented=on  Seed=3244333  SampleTime=ModelParam_noiseGPSSampTime
  Uniform Random Number4 : UniformRandomNumber  Minimum=[-1,-1,-2]  Maximum=[1,1,2]  Seed=[5445,45433,33433]  SampleTime=ModelParam_noiseGPSSampTime
  VeScale : Gain  Gain=1E2
  VelScale : Gain  Gain=1E2
  altScale : Gain  Gain=1E3
  latScale : Gain  Gain=1E7
  lonScale : Gain  Gain=1E7
  MavLinkGPS : Outport  VectorParamsAs1DForOutWhenUnconnected=off
  wires:
  Data Type Conversion8/1 -> Bus Creator/5  "eph"
  Gain8/1 -> Data Type Conversion9/1
  Gain6/1 -> Data Type Conversion8/1
  Data Type Conversion9/1 -> Bus Creator/6  "epv"
  time_usec/1 -> Bus Creator/1  "time_usec"
  latScale/1 -> Data Type Conversion4/1
  lonScale/1 -> Data Type Conversion5/1
  altScale/1 -> Data Type Conversion6/1
  Data Type Conversion4/1 -> Bus Creator/2  "lat"
  Data Type Conversion5/1 -> Bus Creator/3  "lon"
  Data Type Conversion6/1 -> Bus Creator/4  "alt"
  Demux2/1 -> Bus Creator/8  "vn"
  Demux2/2 -> Bus Creator/9  "ve"
  Demux2/3 -> Bus Creator/10  "vd"
  VeScale/1 -> Data Type Conversion3/1
  Data Type Conversion3/1 -> Demux2/1
  VelScale/1 -> Data Type Conversion2/1
  Data Type Conversion2/1 -> Bus Creator/7  "vel"
  AngleScale/1 -> Data Type Conversion7/1
  Data Type Conversion7/1 -> Bus Creator/11  "cog"
  Data Type Conversion11/1 -> Bus Creator/13  "satellites_visible"
  Data Type Conversion10/1 -> Bus Creator/12  "fix_type"
  Demux/1 -> latScale/1
  Demux/2 -> lonScale/1
  Demux/3 -> altScale/1
  Uniform Random Number/1 -> Gain2/1
  ModelParam.GPSEphFinal/1 -> Gain6/1
  Sum2/1 -> Motor_Dynamics_3/1
  Ve/1 -> Sum3/1
  GenCogVel/1(v) -> VelScale/1
  Bus Creator/1 -> MavLinkGPS/1
  BiasGain1/1 -> NoiseFilter1/1(In1)
  Uniform Random Number4/1 -> BiasGain1/1
  GenCogVel/2(cot) -> AngleScale/1
  Sum1/1 -> Motor_Dynamics_1/1
  Uniform Random Number2/1 -> Sum1/2
  Uniform Random Number3/1 -> Sum2/2
  ModelParam.GPSEpvFinal/1 -> Gain8/1
  Sum3/1 -> GenCogVel/1(u), VeScale/1
  NoiseFilter1/1(Out1) -> Sum3/2
  Bus Selector/2 -> Data Type Conversion10/1  "<3DFix>"
  Xe1/1 -> GPSFault/1
  Bus Selector/1 -> Demux/1  "<GPSOut>"
  GPSFault/1 -> Bus Selector/1
  Bus Selector/3 -> Data Type Conversion11/1  "<Sats>"
  [FaultIn] -> GPSFault/2

== system USV/SensorModel/HILSensorMavModel1 ==
  time_usec : Inport
  Gravity : Inport  Port=2
  TempC : Inport  Port=3
  pressure : Inport  Port=4
  GPSPos : Inport  Port=5
  wb : Inport  Port=6
  dwt : Inport  Port=7
  Ab : Inport  Port=8
  DCMbe : Inport  Port=9
  windB : Inport  Port=10
  PWMin : Inport  Port=11
  rho : Inport  Port=12
  Subsystem : Subsystem
  SensorOut : Outport  VectorParamsAs1DForOutWhenUnconnected=off
  MagDeclination : Outport  Port=2  VectorParamsAs1DForOutWhenUnconnected=off
  acc : Outport  Port=3  VectorParamsAs1DForOutWhenUnconnected=off
  wires:
  PWMin/1 -> Subsystem/10(PWMin)
  Subsystem/2(MagDeclination) -> MagDeclination/1
  DCMbe/1 -> Subsystem/9(DCMbe)
  wb/1 -> Subsystem/7(wb)
  Subsystem/1(SensorOut) -> SensorOut/1
  Subsystem/3(acc) -> acc/1
  dwt/1 -> Subsystem/8(dwt)
  rho/1 -> Subsystem/3(rho)
  TempC/1 -> Subsystem/4(TempC)
  windB/1 -> Subsystem/2(windB)
  pressure/1 -> Subsystem/1(pressure)
  time_usec/1 -> Subsystem/11(time_usec)  "time_usec"
  Ab/1 -> Subsystem/6(Ab)
  GPSPos/1 -> Subsystem/5(GPSPos)
  Gravity/1 -> Subsystem/12(Gravity)
